simulink model "Simulink_Model"  (R2021a)
settings: Solver=FixedStepDiscrete  StartTime=0.0  StopTime=inf  FixedStep=1  RelTol=1e-3
settings Model: EnablePacing=on  Creator=matteopenlington  LastModifiedBy=matteopenlington
settings DebuggingCC: UnderSpecifiedDimensionMsg=warning

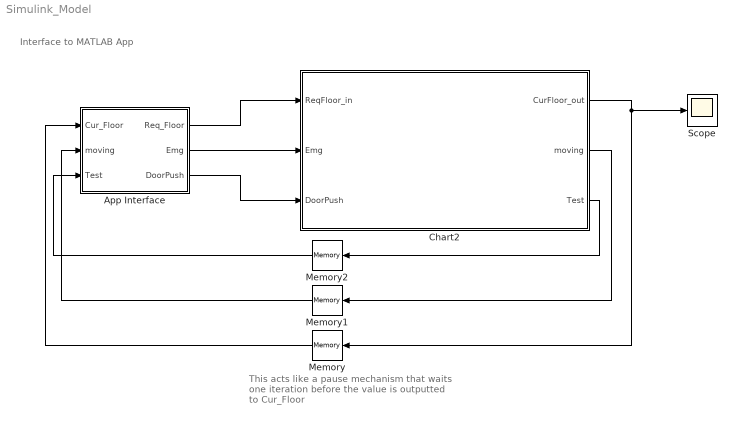
== system Simulink_Model ==
  note: This acts like a pause mechanism that waits one iteration before the value is outputted to Cur_Floor
  note: Interface to MATLAB App
  App Interface : Stateflow chart  TreatAsAtomicUnit=on
  Chart2 : Stateflow chart  TreatAsAtomicUnit=on
  Memory : Memory
  Memory1 : Memory
  Memory2 : Memory
  Scope : Scope
  wires:
  App Interface/1(Req_Floor) -> Chart2/1(ReqFloor_in)
  Memory/1 -> App Interface/1(Cur_Floor)
  Chart2/1(CurFloor_out) -> Scope/1, Memory/1
  App Interface/2(Emg) -> Chart2/2(Emg)
  Chart2/2(moving) -> Memory1/1
  Memory1/1 -> App Interface/2(moving)
  App Interface/3(DoorPush) -> Chart2/3(DoorPush)
  Chart2/3(Test) -> Memory2/1
  Memory2/1 -> App Interface/3(Test)

== stateflow chart Simulink_Model/App Interface ==
  state InterfaceFromApp
    en:
    coder.extrinsic('AppWSimulink', 'updateCounter', 'Logic', 'Emergency', 'DoorOperation', 'updateDoorStatus');
    app = AppWSimulink(this);
    %Req_Floor = 2;
    initialiseData();
    Logic(app,Req_Floor);
    Emergency(app,Emg);
    DoorOperation(app, DoorPush)
    du:
    if hasChanged(Cur_Floor)
    updateCounter(app, Cur_Floor, Test, Req_Floor);
    end
    if isequal(Cur_Floor, Req_Floor)
    updateDoorStatus(app,Test);
    end
    if (Emg == 1)
    Reset;
    end
    state initialiseData [function]
      (default) -> (junction 12) : {
          | %CurFloor = 0;
          | Req_Floor = 0;
          | Emg = 0;
          | DoorPush =0;
          | }
    state Reset [function]
      (default) -> (junction 119) : {
          | Req_Floor = -10;
          | DoorPush =0;
          | }
  (default) -> InterfaceFromApp
  data: app local; Cur_Floor input; Req_Floor output; Emg output; moving input; DoorPush output; Test input

== stateflow chart Simulink_Model/Chart2 ==
  state No_Error1
    entry:
    CurFloor = 0;
    Door = 0;
    hasOpened = 1;
    doorClose = 0;
    state Motion [group]
      state MovingUp
        entry:
        moving = 1;
        CurFloor = CurFloor +1;
        exit:
        moving = 0;
      state MovingDown
        entry:
        moving = 1;
        exit:
        CurFloor = CurFloor - 1;
        moving =0;
    state Not_Moving
      entry:
      CurFloor_out = CurFloor;
      NxtFloor;
      Test = DoorPush;
      state NxtFloor [function]
        (default) -> (junction 99)
        (junction 99) -> (junction 101) [order 1] : [isempty(ReqFloor_in)]{ReqFloor = -10}
        (junction 99) -> (junction 103) [order 2] : {ReqFloor = ReqFloor_in;}
        (junction 101) -> (junction 105)
        (junction 103) -> (junction 105)
      state Idle
        en:
      state Doors
        state DoorOpen
          entry:
          door = 1;
          Test = 1;
          pause(2);
          hasOpened = 1;
        state DoorClose
          entry:
          door = 0;
          Test =0;
          pause(2);
          doorClose = 1;
        DoorClose -> DoorOpen
        DoorOpen -> DoorClose [commented out] : [Sensor == 0 && DoorPush == 1]
        DoorOpen -> DoorClose : [Sensor ==0]
      (default) -> Idle
      Idle -> DoorOpen [order 1] : [ReqFloor == CurFloor && hasOpened == 0]
    (default) -> Not_Moving
    Not_Moving -> MovingUp [order 1] : [ReqFloor > CurFloor]{hasOpened = 0}
    MovingUp -> Not_Moving : after(2,sec)
    Idle -> (junction 180) [order 2]
    (junction 180) -> (junction 177)
    MovingDown -> Not_Moving : after(2,sec)
    (junction 177) -> Not_Moving : after(0.001,sec)
    (junction 182) -> (junction 177)
    Not_Moving -> MovingDown [order 2] : [-2 < ReqFloor && ReqFloor < CurFloor]{hasOpened = 0}
    Doors -> (junction 182) : [doorClose == 1]
  state Emergency
    en:
    Test = 0;
    hasOpened = 0;
  (default) -> No_Error1
  No_Error1 -> Emergency : [Emg == 1]
  Emergency -> No_Error1 : [Emg  == 0]
  data: Door local; Sensor local =0; CurFloor local; ReqFloor_in input; CurFloor_out output; ReqFloor local; Emg input; moving output; DoorPush input; door local; Test output; hasOpened local; doorClose local
